simulink model "quarc_sine_scope"  (R2020a)
settings: Solver=FixedStepDiscrete  StartTime=0.0  StopTime=inf  FixedStep=0.06  RelTol=1e-3  EnableMultiTasking=on
model workspace (MAT data in the model file):
  amplitude = 0
libraries: quarc_library x1
settings Model: SimulationMode=external  ExtModeTrigDuration=10000  Creator=Luis de la Torre  LastModifiedBy=Luis de la Torre
settings SolverCC: PositivePriorityOrder=on
settings DataIOCC: SaveOutput=off  SignalLogging=off  DSMLogging=off  SaveTime=off  ReturnWorkspaceOutputs=off
settings OptimizationCC: LifeSpan=inf
settings DebuggingCC: ArithmeticOperatorsInVariantConditions=warning
settings SFSimCC: SimUseLocalCustomCode=off  CustomCodeUndefinedFunction=UseInterfaceOnly
settings RTWCC: Description=QUARC Win64 Target  SystemTargetFile=quarc_win64.tlc  TemplateMakefile=quarc_default_tmf  RTWVerbose=off  RTWUseLocalCustomCode=off
settings CodeAppCC: StateflowObjectComments=on
settings STFCustomTargetCC: TargetPreCompLibLocation=C:\PROGRA~3\QUARC\lib\2020a\win64\release  TargetLangStandard=C99 (ISO)  ConcurrentExecutionCompliant=on  GRTInterface=on  SystemTargetFile=quarc_win64.tlc
settings GRTTargetCC: TargetPreCompLibLocation=C:\PROGRA~3\QUARC\lib\2020a\win64\release  ParMdlRefBuildCompliant=off  CompOptLevelCompliant=off  CombineOutputUpdateFcns=off  MatFileLogging=off  CPPClassGenCompliant=off  GRTInterface=on  UseToolchainInfoCompliant=off  ExtMode=on  ExtModeMexFile=quarc_comm
settings ConfigComp: CovMetricSettings=dswe

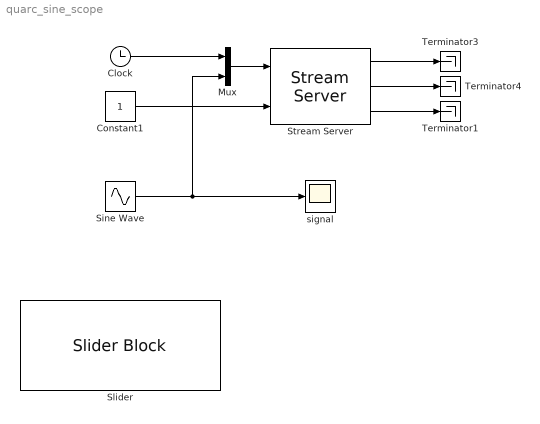
== system quarc_sine_scope ==
  Clock : Clock
      settings: Decimation=100
  Constant1 : Constant  SampleTime=0.06
  Mux : Mux  Inputs=2
  Sine Wave : Sin  Amplitude=amplitude  SampleTime=0.06
  Slider : SliderBlock
  Stream Server : quarc_library/Communications/Basic/Stream Server  uri_source=Specify via dialog (do not evaluate)  uri=tcpip://192.168.137.1:18000?nagle='off'  apply_uri_to_all_configs=on  send_buffer_size=16  receive_buffer_size=1460  byte_order=little endian (Intel - LSB first)  optimization=Minimum latency  send_options=Send most recent data  receive_options=Do not receive data  default_value=[0]  sample_time=qc_get_step_size  active=off  implementation=Use blocking I/O in a separate thread  send_fifo_size=1  receive_fifo_size=1  send_priority=0  receive_priority=2  send_dimensions=off  receive_dimensions=off  max_dimensions=-1  data_type=Inherited via back propagation  type_expr=BusObject
      settings: AttributesFormatString="\"tcpip://192.168.137.1:18000?nagle='off'\""
  Terminator1 : Terminator
  Terminator3 : Terminator
  Terminator4 : Terminator
  signal : Scope
  wires:
  Clock/1 -> Mux/1
  Sine Wave/1 -> Mux/2, signal/1
  Stream Server/2 -> Terminator4/1
  Mux/1 -> Stream Server/1
  Stream Server/3 -> Terminator1/1
  Stream Server/1 -> Terminator3/1
  Constant1/1 -> Stream Server/2
